simulink model "FaultCheck"  (R2022b)
settings: Solver=FixedStepAuto  StartTime=0.0  StopTime=10  FixedStep=1  RelTol=1e-3
undefined symbols (not defined in the file): C_Flt_IGBTULowerTempConfirmTh_u16, C_Flt_IGBTULowerTempDiagEn_b, C_Flt_IGBTULowerTempErrCode_u16, C_Flt_IGBTULowerTempPowerCoeff, C_Flt_IGBTULowerTempRecoveryTh_u16, C_Flt_IGBTULowerTempRecTh_s32, C_Flt_IGBTULowerTempTrigTh_s32, C_Flt_IGBTUOverTempConfirmTh_u16, C_Flt_IGBTUOverTempDiagEn_b, C_Flt_IGBTUOverTempErrCode_u16, C_Flt_IGBTUOverTempRecoveryTh_u16, C_Flt_IGBTUOverTempRecTh_s32, C_Flt_IGBTUOverTempTrigTh_s32, C_Flt_IGBTVLowerTempConfirmTh_u16, C_Flt_IGBTVLowerTempDiagEn_b, C_Flt_IGBTVLowerTempErrCode_u16, C_Flt_IGBTVLowerTempPowerCoeff, C_Flt_IGBTVLowerTempRecoveryTh_u16, C_Flt_IGBTVLowerTempRecTh_s32, C_Flt_IGBTVLowerTempTrigTh_s32, C_Flt_IGBTVOverTempConfirmTh_u16, C_Flt_IGBTVOverTempDiagEn_b, C_Flt_IGBTVOverTempErrCode_u16, C_Flt_IGBTVOverTempRecoveryTh_u16, C_Flt_IGBTVOverTempRecTh_s32, C_Flt_IGBTVOverTempTrigTh_s32, C_Flt_IGBTWLowerTempConfirmTh_u16, C_Flt_IGBTWLowerTempDiagEn_b, C_Flt_IGBTWLowerTempErrCode_u16, C_Flt_IGBTWLowerTempPowerCoeff, C_Flt_IGBTWLowerTempRecoveryTh_u16, C_Flt_IGBTWLowerTempRecTh_s32, C_Flt_IGBTWLowerTempTrigTh_s32, C_Flt_IGBTWOverTempConfirmTh_u16, C_Flt_IGBTWOverTempDiagEn_b, C_Flt_IGBTWOverTempErrCode_u16, C_Flt_IGBTWOverTempRecoveryTh_u16, C_Flt_IGBTWOverTempRecTh_s32, C_Flt_IGBTWOverTempTrigTh_s32, C_Flt_IuOCConfirmTh_u16, C_Flt_IuOCDiagEn_b, C_Flt_IuOCErrCode_u16, C_Flt_IuOCNegLimit_s32, C_Flt_IuOCPosLimit_s32, C_Flt_IuOCRecoveryTh_u16, C_Flt_IuZeroDriftDiagEn_b, C_Flt_IuZeroDriftErrCode_u16, C_Flt_IvOCConfirmTh_u16, C_Flt_IvOCDiagEn_b, C_Flt_IvOCErrCode_u16, C_Flt_IvOCNegLimit_s32, C_Flt_IvOCPosLimit_s32, C_Flt_IvOCRecoveryTh_u16, C_Flt_IvZeroDriftDiagEn_b, C_Flt_IvZeroDriftErrCode_u16, C_Flt_IwOCConfirmTh_u16, C_Flt_IwOCDiagEn_b, C_Flt_IwOCErrCode_u16, C_Flt_IwOCNegLimit_s32, C_Flt_IwOCPosLimit_s32 ... (+196)
libraries: YS_UserDefined_Library x21, simulink x5
(part 6 of 11)

== system FaultCheck/FaultDiagnose/UdcLowerTwoDiag/Diagnose/Disable ==
  Action Port : ActionPort  ActionPortLabel=if(u1 == 0)
  Constant : Constant  Value=C_Flt_NoErr_b
  UdcLowerTwoFltDeb : Outport
  wires:
  Constant/1 -> UdcLowerTwoFltDeb/1

== system FaultCheck/FaultDiagnose/UdcLowerTwoDiag/Diagnose/NormalDiag ==
  Udc : Inport
  Parameter : Inport  Port=2
  Action Port : ActionPort  ActionPortLabel=else
  Bus Selector : BusSelector  OutputSignals=UdcLowerTwoConfirmTh,UdcLowerTwoRecoveryTh,UdcLowerTwoTrigTh,UdcLowerTwoRecTh
  DebounceRecInTwo : YS_UserDefined_Library/Fault/DebounceRecInTwo  SystemSampleTime=-1  VariantActivationTime=update diagram  Latency=0  AutoFrameSizeCalculation=off
      settings: SourceProductName=YS
  Relational Operator : RelationalOperator  Operator=>  OutDataTypeStr=boolean  RndMeth=Simplest  InputSameDT=off
  Relational Operator1 : RelationalOperator  Operator=>  OutDataTypeStr=boolean  RndMeth=Simplest  InputSameDT=off
  Signal Copy : SignalConversion  OverrideOpt=off
  UdcLowerTwoFltDeb : Outport
  wires:
  Parameter/1 -> Bus Selector/1
  Bus Selector/1 -> DebounceRecInTwo/1  "<UdcLowerTwoConfirmTh>"
  Bus Selector/2 -> DebounceRecInTwo/2  "<UdcLowerTwoRecoveryTh>"
  DebounceRecInTwo/1 -> Signal Copy/1  "M_Flt_UdcLowerTwoFltFlgDeb_b"
  Relational Operator/1 -> DebounceRecInTwo/3  "M_Flt_UdcLowerTwoFltFlgUnDeb_b"
  Signal Copy/1 -> UdcLowerTwoFltDeb/1
  Bus Selector/3 -> Relational Operator/1  "<UdcLowerTwoTrigTh>"
  Udc/1 -> Relational Operator/2, Relational Operator1/1
  Bus Selector/4 -> Relational Operator1/2  "<UdcLowerTwoRecTh>"
  Relational Operator1/1 -> DebounceRecInTwo/4  "M_Flt_UdcLowerTwoRecFlgUnDeb_b"

== system FaultCheck/FaultDiagnose/UdcLowerTwoDiag/FaultLevelDeter/LowerTwo ==
  FaultLevel : Inport
  Action Port : ActionPort  ActionPortLabel=else
  UdcLowerTwoFltLevel : Outport
  wires:
  FaultLevel/1 -> UdcLowerTwoFltLevel/1

== system FaultCheck/FaultDiagnose/UdcLowerTwoDiag/FaultLevelDeter/Normal ==
  Action Port : ActionPort  ActionPortLabel=if(u1 == 0)
  Constant : Constant  Value=C_Flt_LevelZero_u8
  UdcLowerTwoFltLevel : Outport
  wires:
  Constant/1 -> UdcLowerTwoFltLevel/1

== system FaultCheck/FaultDiagnose/UdcLowerTwoDiag/PowerReductionCoeffDeter/If Action Subsystem ==
  Action Port : ActionPort  ActionPortLabel=if(u1 < 2)
  Constant : Constant  Value=C_Flt_PowerCoeffOne_s32
  Coeff : Outport
  wires:
  Constant/1 -> Coeff/1

== system FaultCheck/FaultDiagnose/UdcLowerTwoDiag/PowerReductionCoeffDeter/If Action Subsystem1 ==
  PowerCoeff : Inport
  Action Port : ActionPort  ActionPortLabel=elseif(u1 == 2)
  Coeff : Outport
  wires:
  PowerCoeff/1 -> Coeff/1

== system FaultCheck/FaultDiagnose/UdcLowerTwoDiag/PowerReductionCoeffDeter/If Action Subsystem2 ==
  Action Port : ActionPort  ActionPortLabel=else
  Constant : Constant  Value=C_Flt_PowerCoeffZero_s32
  Coeff : Outport
  wires:
  Constant/1 -> Coeff/1

== system FaultCheck/FaultDiagnose/UdcOverOneDiag/Diagnose/Disable ==
  Action Port : ActionPort  ActionPortLabel=if(u1 == 0)
  Constant : Constant  Value=C_Flt_NoErr_b
  UdcOverOneFltDeb : Outport
  wires:
  Constant/1 -> UdcOverOneFltDeb/1

== system FaultCheck/FaultDiagnose/UdcOverOneDiag/Diagnose/NormalDiag ==
  Udc : Inport
  Parameter : Inport  Port=2
  Action Port : ActionPort  ActionPortLabel=else
  Bus Selector : BusSelector  OutputSignals=UdcOverOneConfirmTh,UdcOverOneRecoveryTh,UdcOverOneTrigTh,UdcOverOneRecTh
  DebounceRecInTwo : YS_UserDefined_Library/Fault/DebounceRecInTwo  SystemSampleTime=-1  VariantActivationTime=update diagram  Latency=0  AutoFrameSizeCalculation=off
      settings: SourceProductName=YS
  Relational Operator : RelationalOperator  Operator=<  OutDataTypeStr=boolean  RndMeth=Simplest  InputSameDT=off
  Relational Operator1 : RelationalOperator  Operator=<  OutDataTypeStr=boolean  RndMeth=Simplest  InputSameDT=off
  Signal Copy : SignalConversion  OverrideOpt=off
  UdcOverOneFltDeb : Outport
  wires:
  Parameter/1 -> Bus Selector/1
  Bus Selector/1 -> DebounceRecInTwo/1  "<UdcOverOneConfirmTh>"
  Bus Selector/2 -> DebounceRecInTwo/2  "<UdcOverOneRecoveryTh>"
  DebounceRecInTwo/1 -> Signal Copy/1  "M_Flt_UdcOverOneFltFlgDeb_b"
  Relational Operator/1 -> DebounceRecInTwo/3  "M_Flt_UdcOverOneFltFlgUnDeb_b"
  Signal Copy/1 -> UdcOverOneFltDeb/1
  Bus Selector/3 -> Relational Operator/1  "<UdcOverOneTrigTh>"
  Udc/1 -> Relational Operator1/1, Relational Operator/2
  Bus Selector/4 -> Relational Operator1/2  "<UdcOverOneRecTh>"
  Relational Operator1/1 -> DebounceRecInTwo/4  "M_Flt_UdcOverOneRecFlgUnDeb_b"

== system FaultCheck/FaultDiagnose/UdcOverOneDiag/FaultLevelDeter/Normal ==
  Action Port : ActionPort  ActionPortLabel=if(u1 == 0)
  Constant : Constant  Value=C_Flt_LevelZero_u8
  UdcOverOneFltLevel : Outport
  wires:
  Constant/1 -> UdcOverOneFltLevel/1

== system FaultCheck/FaultDiagnose/UdcOverOneDiag/FaultLevelDeter/OverOne ==
  FaultLevel : Inport
  Action Port : ActionPort  ActionPortLabel=else
  UdcOverOneFltLevel : Outport
  wires:
  FaultLevel/1 -> UdcOverOneFltLevel/1

== system FaultCheck/FaultDiagnose/UdcOverOneDiag/PowerReductionCoeffDeter/If Action Subsystem ==
  Action Port : ActionPort  ActionPortLabel=if(u1 < 2)
  Constant : Constant  Value=C_Flt_PowerCoeffOne_s32
  Coeff : Outport
  wires:
  Constant/1 -> Coeff/1

== system FaultCheck/FaultDiagnose/UdcOverOneDiag/PowerReductionCoeffDeter/If Action Subsystem1 ==
  PowerCoeff : Inport
  Action Port : ActionPort  ActionPortLabel=elseif(u1 == 2)
  Coeff : Outport
  wires:
  PowerCoeff/1 -> Coeff/1

== system FaultCheck/FaultDiagnose/UdcOverOneDiag/PowerReductionCoeffDeter/If Action Subsystem2 ==
  Action Port : ActionPort  ActionPortLabel=else
  Constant : Constant  Value=C_Flt_PowerCoeffZero_s32
  Coeff : Outport
  wires:
  Constant/1 -> Coeff/1

== system FaultCheck/FaultDiagnose/UdcOverTwoDiag/Diagnose/Disable ==
  Action Port : ActionPort  ActionPortLabel=if(u1 == 0)
  Constant : Constant  Value=C_Flt_NoErr_b
  UdcOverTwoFltDeb : Outport
  wires:
  Constant/1 -> UdcOverTwoFltDeb/1

== system FaultCheck/FaultDiagnose/UdcOverTwoDiag/Diagnose/NormalDiag ==
  Udc : Inport
  Parameter : Inport  Port=2
  Action Port : ActionPort  ActionPortLabel=else
  Bus Selector : BusSelector  OutputSignals=UdcOverTwoConfirmTh,UdcOverTwoRecoveryTh,UdcOverTwoTrigTh
  DebounceUnRec1 : YS_UserDefined_Library/Fault/DebounceUnRec  SystemSampleTime=-1  VariantActivationTime=update diagram  Latency=0  AutoFrameSizeCalculation=off
      settings: SourceProductName=YS
  Relational Operator : RelationalOperator  Operator=<  OutDataTypeStr=boolean  RndMeth=Simplest  InputSameDT=off
  Signal Copy : SignalConversion  OverrideOpt=off
  UdcOverTwoFltDeb : Outport
  wires:
  Parameter/1 -> Bus Selector/1
  Bus Selector/1 -> DebounceUnRec1/1  "<UdcOverTwoConfirmTh>"
  Bus Selector/2 -> DebounceUnRec1/2  "<UdcOverTwoRecoveryTh>"
  DebounceUnRec1/1 -> Signal Copy/1  "M_Flt_UdcOverTwoFltFlgDeb_b"
  Relational Operator/1 -> DebounceUnRec1/3  "M_Flt_UdcOverTwoFltFlgUnDeb_b"
  Signal Copy/1 -> UdcOverTwoFltDeb/1
  Bus Selector/3 -> Relational Operator/1  "<UdcOverTwoTrigTh>"
  Udc/1 -> Relational Operator/2

== system FaultCheck/FaultDiagnose/UdcOverTwoDiag/FaultLevelDeter/Normal ==
  Action Port : ActionPort  ActionPortLabel=if(u1 == 0)
  Constant : Constant  Value=C_Flt_LevelZero_u8
  UdcOverTwoFltLevel : Outport
  wires:
  Constant/1 -> UdcOverTwoFltLevel/1

== system FaultCheck/FaultDiagnose/UdcOverTwoDiag/FaultLevelDeter/OverTwo ==
  FaultLevel : Inport
  Action Port : ActionPort  ActionPortLabel=else
  UdcOverTwoFltLevel : Outport
  wires:
  FaultLevel/1 -> UdcOverTwoFltLevel/1

== system FaultCheck/FaultDiagnose/UdcOverTwoDiag/PowerReductionCoeffDeter/If Action Subsystem ==
  Action Port : ActionPort  ActionPortLabel=if(u1 < 2)
  Constant : Constant  Value=C_Flt_PowerCoeffOne_s32
  Coeff : Outport
  wires:
  Constant/1 -> Coeff/1

== system FaultCheck/FaultDiagnose/UdcOverTwoDiag/PowerReductionCoeffDeter/If Action Subsystem1 ==
  PowerCoeff : Inport
  Action Port : ActionPort  ActionPortLabel=elseif(u1 == 2)
  Coeff : Outport
  wires:
  PowerCoeff/1 -> Coeff/1

== system FaultCheck/FaultDiagnose/UdcOverTwoDiag/PowerReductionCoeffDeter/If Action Subsystem2 ==
  Action Port : ActionPort  ActionPortLabel=else
  Constant : Constant  Value=C_Flt_PowerCoeffZero_s32
  Coeff : Outport
  wires:
  Constant/1 -> Coeff/1

== system FaultCheck/FltCheck/Determination/Detection Criteria/Determination ==
  Condition : Inport
  EQ : Inport  Port=2
  GT : Inport  Port=3
  LT : Inport  Port=4
  NEQ : Inport  Port=5
  Multiport Switch : MultiPortSwitch  Inputs=4  SaturateOnIntegerOverflow=off  InputSameDT=off
  Fail : Outport
  wires:
  EQ/1 -> Multiport Switch/2
  GT/1 -> Multiport Switch/3
  LT/1 -> Multiport Switch/4
  NEQ/1 -> Multiport Switch/5
  Condition/1 -> Multiport Switch/1
  Multiport Switch/1 -> Fail/1

== system FaultCheck/FltCheck/Determination/Detection Criteria/Equal ==
  FltSrc : Inport
  FltTh : Inport  Port=2
  Constant : Constant  OutDataTypeStr=boolean
  Constant1 : Constant  Value=0  OutDataTypeStr=boolean
  Relational Operator : RelationalOperator  Operator===  OutDataTypeStr=boolean  RndMeth=Simplest  InputSameDT=off
  Switch : Switch  Criteria=u2 ~= 0  SaturateOnIntegerOverflow=off  InputSameDT=off
  EQ : Outport
  wires:
  FltSrc/1 -> Relational Operator/1
  FltTh/1 -> Relational Operator/2
  Relational Operator/1 -> Switch/2
  Constant/1 -> Switch/1
  Constant1/1 -> Switch/3
  Switch/1 -> EQ/1

== system FaultCheck/FltCheck/Determination/Detection Criteria/Lower ==
  FltSrc : Inport
  FltTh : Inport  Port=2
  Constant : Constant  OutDataTypeStr=boolean
  Constant1 : Constant  Value=0  OutDataTypeStr=boolean
  Relational Operator : RelationalOperator  Operator=<  OutDataTypeStr=boolean  RndMeth=Simplest  InputSameDT=off
  Switch : Switch  Criteria=u2 ~= 0  SaturateOnIntegerOverflow=off  InputSameDT=off
  LT : Outport
  wires:
  FltSrc/1 -> Relational Operator/1
  FltTh/1 -> Relational Operator/2
  Relational Operator/1 -> Switch/2
  Constant/1 -> Switch/1
  Constant1/1 -> Switch/3
  Switch/1 -> LT/1

== system FaultCheck/FltCheck/Determination/Detection Criteria/NotEqual ==
  FltSrc : Inport
  FltTh : Inport  Port=2
  Constant : Constant  OutDataTypeStr=boolean
  Constant1 : Constant  Value=0  OutDataTypeStr=boolean
  Relational Operator : RelationalOperator  Operator=~=  OutDataTypeStr=boolean  RndMeth=Simplest  InputSameDT=off
  Switch : Switch  Criteria=u2 ~= 0  SaturateOnIntegerOverflow=off  InputSameDT=off
  NEQ : Outport
  wires:
  Switch/1 -> NEQ/1
  Constant1/1 -> Switch/3
  Constant/1 -> Switch/1
  Relational Operator/1 -> Switch/2
  FltTh/1 -> Relational Operator/2
  FltSrc/1 -> Relational Operator/1

== system FaultCheck/FltCheck/Determination/Detection Criteria/Overflow ==
  FltSrc : Inport
  FltTh : Inport  Port=2
  Constant : Constant  OutDataTypeStr=boolean
  Constant1 : Constant  Value=0  OutDataTypeStr=boolean
  Relational Operator : RelationalOperator  Operator=>  OutDataTypeStr=boolean  RndMeth=Simplest  InputSameDT=off
  Switch : Switch  Criteria=u2 ~= 0  SaturateOnIntegerOverflow=off  InputSameDT=off
  GT : Outport
  wires:
  Switch/1 -> GT/1
  Constant1/1 -> Switch/3
  Constant/1 -> Switch/1
  Relational Operator/1 -> Switch/2
  FltTh/1 -> Relational Operator/2
  FltSrc/1 -> Relational Operator/1

== system FaultCheck/FaultDiag_HighTask_100us/FltDetn/CurrentSensorDetn/Flt_CurrentSensorDetn/ErrCode ==
  note: SWFD--ComReq-01-13
  ErrDetnFlgOut : Inport
  ErrCode : Inport  Port=2
  If : If  IfExpression=u1==0
  If Action Subsystem : Subsystem  TreatAsAtomicUnit=on
  If Action Subsystem1 : Subsystem  TreatAsAtomicUnit=on
  wires:
  ErrCode/1 -> If Action Subsystem1/1(ErrCod)
  If/1 -> If Action Subsystem/Action
  If/2 -> If Action Subsystem1/Action
  ErrDetnFlgOut/1 -> If/1

== system FaultCheck/FaultDiag_HighTask_100us/FltDetn/CurrentSensorDetn/Flt_CurrentSensorDetn/ErrDetn ==
  InputVal : Inport
  EnabDetn : Inport  Port=2
  ActvnDetn : Inport  Port=3
  ErrDeb : Inport  Port=4
  AND1 : Logic  AllPortsSameDT=off  OutDataTypeStr=boolean
  Constant10 : Constant  Value=FLT_ON
  Constant9 : Constant  Value=FLT_ON
  If : If  IfExpression=u1 == 0
  If Action Subsystem : Subsystem  TreatAsAtomicUnit=on
  If Action Subsystem1 : Subsystem  TreatAsAtomicUnit=on
  Merge : Merge
  Relational Operator3 : RelationalOperator  Operator===  OutDataTypeStr=boolean  RndMeth=Simplest  InputSameDT=off
  Relational Operator4 : RelationalOperator  Operator===  OutDataTypeStr=boolean  RndMeth=Simplest  InputSameDT=off
  Flt_CurrentSensorErrFlg : Outport
  wires:
  InputVal/1 -> If Action Subsystem1/1(InputVal)
  ActvnDetn/1 -> Relational Operator3/1
  Constant10/1 -> Relational Operator4/1
  EnabDetn/1 -> Relational Operator4/2
  Relational Operator3/1 -> AND1/1
  Constant9/1 -> Relational Operator3/2
  Relational Operator4/1 -> AND1/2
  AND1/1 -> If/1
  If/1 -> If Action Subsystem/Action
  If/2 -> If Action Subsystem1/Action
  If Action Subsystem1/1(Out1) -> Merge/2
  If Action Subsystem/1(Out1) -> Merge/1
  Merge/1 -> Flt_CurrentSensorErrFlg/1
  ErrDeb/1 -> If Action Subsystem1/2(ErrDeb)

== system FaultCheck/FaultDiag_HighTask_100us/FltDetn/CurrentSensorDetn/Flt_CurrentSensorDetn/FltLvl ==
  note: SWFD--ComReq-01-09
      | SWFD--ComReq-01-10
      | SWFD--ComReq-01-11
      | SWFD--ComReq-01-12
  ErrDetnFlgOut : Inport
  FltLvl : Inport  Port=2
  If : If  IfExpression=u1==0
  If Action Subsystem : Subsystem  TreatAsAtomicUnit=on
  If Action Subsystem1 : Subsystem  TreatAsAtomicUnit=on
  Merge : Merge
  Flt_CurrentSensorFltLvl : Outport
  wires:
  If Action Subsystem/1(ValOut) -> Merge/1
  Merge/1 -> Flt_CurrentSensorFltLvl/1  "Flt_CurrentSensorFltLvl"
  If/1 -> If Action Subsystem/Action
  If/2 -> If Action Subsystem1/Action
  ErrDetnFlgOut/1 -> If/1
  FltLvl/1 -> If Action Subsystem1/1(In)
  If Action Subsystem1/1(ValOut) -> Merge/2

== system FaultCheck/FaultDiag_HighTask_100us/FltDetn/CurrentSensorDetn/Flt_CurrentSensorDetn/Power Reduction Coefficient ==
  note: SWFD--ComReq-01-06
      | SWFD--ComReq-01-07
      | SWFD--ComReq-01-08
      | SWFD--ComReq-01-09
  FltLvlOut : Inport
  PowRecCoef : Inport  Port=2
  If : If  IfExpression=u1<2  ElseIfExpressions=u1==2
  If Action Subsystem : Subsystem  TreatAsAtomicUnit=on
  If Action Subsystem1 : Subsystem  TreatAsAtomicUnit=on
  If Action Subsystem2 : Subsystem  TreatAsAtomicUnit=on
  Merge : Merge  Inputs=3
  Flt_CurrentSensorPowRecCoefOut : Outport
  wires:
  If/1 -> If Action Subsystem/Action
  If Action Subsystem2/1(PowRecCoefOut) -> Merge/3
  If/3 -> If Action Subsystem2/Action
  FltLvlOut/1 -> If/1
  PowRecCoef/1 -> If Action Subsystem1/1(PowRecCoef)
  If Action Subsystem1/1(PowRecCoefOut) -> Merge/2
  If Action Subsystem/1(PowRecCoefOut) -> Merge/1
  Merge/1 -> Flt_CurrentSensorPowRecCoefOut/1  "Flt_CurrentSensorPowRecCoefOut"
  If/2 -> If Action Subsystem1/Action

== system FaultCheck/FaultDiag_HighTask_100us/FltDetn/CurrentSensorDetn/Flt_CurrentSensorDetn/Subsystem ==
  note: SWFD--ComReq-01-14
  Flt_CurrentSensorErrDetnFlg : Inport
  IPC_IuRaw_A : Inport  Port=2
  IPC_IvRaw_A : Inport  Port=3
  Constant : Constant  Value=Flt_IuCurrentSensorSubValue
  Constant1 : Constant  Value=Flt_IvCurrentSensorSubValue
  Switch : Switch  Criteria=u2 > Threshold  SaturateOnIntegerOverflow=off  InputSameDT=off
  Switch1 : Switch  Criteria=u2 > Threshold  SaturateOnIntegerOverflow=off  InputSameDT=off
  Flt_IuCurrentSensorFin : Outport
  Flt_IvCurrentSensorFin : Outport  Port=2
  wires:
  Switch1/1 -> Flt_IvCurrentSensorFin/1
  Flt_CurrentSensorErrDetnFlg/1 -> Switch/2, Switch1/2
  Constant1/1 -> Switch1/1
  IPC_IvRaw_A/1 -> Switch1/3
  Constant/1 -> Switch/1
  Switch/1 -> Flt_IuCurrentSensorFin/1
  IPC_IuRaw_A/1 -> Switch/3

== system FaultCheck/FaultDiag_HighTask_100us/FltDetn/CurrentZeroDrfDetn/CurrZeroDrfDetn/ErrCode1 ==
  ErrDetnFlgOut : Inport
  ErrCode : Inport  Port=2
  If : If  IfExpression=u1==0
  If Action Subsystem : Subsystem  TreatAsAtomicUnit=on
  If Action Subsystem1 : Subsystem  TreatAsAtomicUnit=on
  wires:
  ErrDetnFlgOut/1 -> If/1
  If/2 -> If Action Subsystem1/Action
  If/1 -> If Action Subsystem/Action
  ErrCode/1 -> If Action Subsystem1/1(ErrCod)

== system FaultCheck/FaultDiag_HighTask_100us/FltDetn/CurrentZeroDrfDetn/CurrZeroDrfDetn/ErrDetn ==
  InputVal : Inport
  EnabDetn : Inport  Port=2
  ActvnDetn : Inport  Port=3
  AND1 : Logic  AllPortsSameDT=off  OutDataTypeStr=boolean
  Constant10 : Constant  Value=FLT_ON
  Constant9 : Constant  Value=FLT_ON
  If : If  IfExpression=u1 == 0
  If Action Subsystem : Subsystem  TreatAsAtomicUnit=on
  If Action Subsystem1 : Subsystem  TreatAsAtomicUnit=on
  Merge : Merge
  Relational Operator3 : RelationalOperator  Operator===  OutDataTypeStr=boolean  RndMeth=Simplest  InputSameDT=off
  Relational Operator4 : RelationalOperator  Operator===  OutDataTypeStr=boolean  RndMeth=Simplest  InputSameDT=off
  Flt_CurrZeroDrfErrFlg : Outport
  wires:
  ActvnDetn/1 -> Relational Operator3/1
  Constant10/1 -> Relational Operator4/1
  EnabDetn/1 -> Relational Operator4/2
  Relational Operator3/1 -> AND1/1
  Constant9/1 -> Relational Operator3/2
  Relational Operator4/1 -> AND1/2
  AND1/1 -> If/1
  If/1 -> If Action Subsystem/Action
  If/2 -> If Action Subsystem1/Action
  If Action Subsystem1/1(Out1) -> Merge/2
  If Action Subsystem/1(Out1) -> Merge/1
  Merge/1 -> Flt_CurrZeroDrfErrFlg/1  "Flt_CurrZeroDrfErrFlg"
  InputVal/1 -> If Action Subsystem1/1(InputVal)

== system FaultCheck/FaultDiag_HighTask_100us/FltDetn/CurrentZeroDrfDetn/CurrZeroDrfDetn/FltLvl ==
  ErrDetnFlgOut : Inport
  FltLvl : Inport  Port=2
  If : If  IfExpression=u1==0
  If Action Subsystem : Subsystem  TreatAsAtomicUnit=on
  If Action Subsystem1 : Subsystem  TreatAsAtomicUnit=on
  Merge : Merge
  Flt_CurrZeroDrfFltLvl : Outport
  wires:
  If Action Subsystem/1(ValOut) -> Merge/1
  Merge/1 -> Flt_CurrZeroDrfFltLvl/1  "Flt_CurrZeroDrfFltLv"
  If/1 -> If Action Subsystem/Action
  If/2 -> If Action Subsystem1/Action
  ErrDetnFlgOut/1 -> If/1
  FltLvl/1 -> If Action Subsystem1/1(In)
  If Action Subsystem1/1(ValOut) -> Merge/2

== system FaultCheck/FaultDiag_HighTask_100us/FltDetn/CurrentZeroDrfDetn/CurrZeroDrfDetn/Power Reduction Coefficient ==
  FltLvlOut : Inport
  PowRecCoef : Inport  Port=2
  If : If  IfExpression=u1<2  ElseIfExpressions=u1==2
  If Action Subsystem : Subsystem  TreatAsAtomicUnit=on
  If Action Subsystem1 : Subsystem  TreatAsAtomicUnit=on
  If Action Subsystem2 : Subsystem  TreatAsAtomicUnit=on
  Merge : Merge  Inputs=3
  Flt_CurrZeroDrfPowRecCoefOut : Outport
  wires:
  If/2 -> If Action Subsystem1/Action
  Merge/1 -> Flt_CurrZeroDrfPowRecCoefOut/1  "Flt_CurrZeroDrfPowRecCoefOut"
  If Action Subsystem/1(PowRecCoefOut) -> Merge/1
  If Action Subsystem1/1(PowRecCoefOut) -> Merge/2
  PowRecCoef/1 -> If Action Subsystem1/1(PowRecCoef)
  FltLvlOut/1 -> If/1
  If/3 -> If Action Subsystem2/Action
  If Action Subsystem2/1(PowRecCoefOut) -> Merge/3
  If/1 -> If Action Subsystem/Action

== system FaultCheck/FaultDiag_HighTask_100us/FltDetn/DriveUdcDetn/DriveUdcDetn/ErrCode ==
  ErrDetnFlgOut : Inport
  ErrCode : Inport  Port=2
  If : If  IfExpression=u1==0
  If Action Subsystem : Subsystem  TreatAsAtomicUnit=on
  If Action Subsystem1 : Subsystem  TreatAsAtomicUnit=on
  wires:
  ErrDetnFlgOut/1 -> If/1
  If/2 -> If Action Subsystem1/Action
  If/1 -> If Action Subsystem/Action
  ErrCode/1 -> If Action Subsystem1/1(ErrCod)

== system FaultCheck/FaultDiag_HighTask_100us/FltDetn/DriveUdcDetn/DriveUdcDetn/ErrDetn ==
  InputVal : Inport
  EnabDetn : Inport  Port=2
  ActvnDetn : Inport  Port=3
  ErrDeb : Inport  Port=4
  AND1 : Logic  AllPortsSameDT=off  OutDataTypeStr=boolean
  Constant10 : Constant  Value=FLT_ON
  Constant9 : Constant  Value=FLT_ON
  If : If  IfExpression=u1 == 0
  If Action Subsystem : Subsystem  TreatAsAtomicUnit=on
  If Action Subsystem1 : Subsystem  TreatAsAtomicUnit=on
  Merge : Merge
  Relational Operator3 : RelationalOperator  Operator===  OutDataTypeStr=boolean  RndMeth=Simplest  InputSameDT=off
  Relational Operator4 : RelationalOperator  Operator===  OutDataTypeStr=boolean  RndMeth=Simplest  InputSameDT=off
  Flt_DriveUdcErrFlg : Outport
  wires:
  ErrDeb/1 -> If Action Subsystem1/2(ErrDeb)
  Merge/1 -> Flt_DriveUdcErrFlg/1  "Flt_DriveUdcErrFlg"
  If Action Subsystem/1(Out1) -> Merge/1
  If Action Subsystem1/1(Out1) -> Merge/2
  If/2 -> If Action Subsystem1/Action
  If/1 -> If Action Subsystem/Action
  AND1/1 -> If/1
  Relational Operator4/1 -> AND1/2
  Constant9/1 -> Relational Operator3/2
  Relational Operator3/1 -> AND1/1
  EnabDetn/1 -> Relational Operator4/2
  Constant10/1 -> Relational Operator4/1
  ActvnDetn/1 -> Relational Operator3/1
  InputVal/1 -> If Action Subsystem1/1(InputVal)

== system FaultCheck/FaultDiag_HighTask_100us/FltDetn/DriveUdcDetn/DriveUdcDetn/FltLvl ==
  ErrDetnFlgOut : Inport
  FltLvl : Inport  Port=2
  If : If  IfExpression=u1==0
  If Action Subsystem : Subsystem  TreatAsAtomicUnit=on
  If Action Subsystem1 : Subsystem  TreatAsAtomicUnit=on
  Merge : Merge
  Flt_DriveUdcFltLvl : Outport
  wires:
  If Action Subsystem1/1(ValOut) -> Merge/2
  FltLvl/1 -> If Action Subsystem1/1(In)
  ErrDetnFlgOut/1 -> If/1
  If/2 -> If Action Subsystem1/Action
  If/1 -> If Action Subsystem/Action
  Merge/1 -> Flt_DriveUdcFltLvl/1  "Flt_DriveUdcFltLvl"
  If Action Subsystem/1(ValOut) -> Merge/1

== system FaultCheck/FaultDiag_HighTask_100us/FltDetn/DriveUdcDetn/DriveUdcDetn/Power Reduction Coefficient ==
  FltLvlOut : Inport
  PowRecCoef : Inport  Port=2
  If : If  IfExpression=u1<2  ElseIfExpressions=u1==2
  If Action Subsystem : Subsystem  TreatAsAtomicUnit=on
  If Action Subsystem1 : Subsystem  TreatAsAtomicUnit=on
  If Action Subsystem2 : Subsystem  TreatAsAtomicUnit=on
  Merge : Merge  Inputs=3
  Flt_DriveUdcPowRecCoefOut : Outport
  wires:
  If/2 -> If Action Subsystem1/Action
  Merge/1 -> Flt_DriveUdcPowRecCoefOut/1  "Flt_DriveUdcPowRecCoefOut"
  If Action Subsystem/1(PowRecCoefOut) -> Merge/1
  If Action Subsystem1/1(PowRecCoefOut) -> Merge/2
  PowRecCoef/1 -> If Action Subsystem1/1(PowRecCoef)
  FltLvlOut/1 -> If/1
  If/3 -> If Action Subsystem2/Action
  If Action Subsystem2/1(PowRecCoefOut) -> Merge/3
  If/1 -> If Action Subsystem/Action

== system FaultCheck/FaultDiag_HighTask_100us/FltDetn/Drive_H_Detn/Drive_H_Detn/ErrCode ==
  ErrDetnFlgOut : Inport
  ErrCode : Inport  Port=2
  If : If  IfExpression=u1==0
  If Action Subsystem : Subsystem  TreatAsAtomicUnit=on
  If Action Subsystem1 : Subsystem  TreatAsAtomicUnit=on
  wires:
  ErrDetnFlgOut/1 -> If/1
  If/2 -> If Action Subsystem1/Action
  If/1 -> If Action Subsystem/Action
  ErrCode/1 -> If Action Subsystem1/1(ErrCod)

== system FaultCheck/FaultDiag_HighTask_100us/FltDetn/Drive_H_Detn/Drive_H_Detn/ErrDetn ==
  InputVal : Inport
  EnabDetn : Inport  Port=2
  ActvnDetn : Inport  Port=3
  ErrDeb : Inport  Port=4
  AND1 : Logic  AllPortsSameDT=off  OutDataTypeStr=boolean
  Constant10 : Constant  Value=FLT_ON
  Constant9 : Constant  Value=FLT_ON
  If : If  IfExpression=u1 == 0
  If Action Subsystem : Subsystem  TreatAsAtomicUnit=on
  If Action Subsystem1 : Subsystem  TreatAsAtomicUnit=on
  Merge : Merge
  Relational Operator3 : RelationalOperator  Operator===  OutDataTypeStr=boolean  RndMeth=Simplest  InputSameDT=off
  Relational Operator4 : RelationalOperator  Operator===  OutDataTypeStr=boolean  RndMeth=Simplest  InputSameDT=off
  Flt_Drive_H_ErrFlg : Outport
  wires:
  ErrDeb/1 -> If Action Subsystem1/2(ErrDeb)
  Merge/1 -> Flt_Drive_H_ErrFlg/1  "Flt_Drive_H_ErrFlg"
  If Action Subsystem/1(Out1) -> Merge/1
  If Action Subsystem1/1(Out1) -> Merge/2
  If/2 -> If Action Subsystem1/Action
  If/1 -> If Action Subsystem/Action
  AND1/1 -> If/1
  Relational Operator4/1 -> AND1/2
  Constant9/1 -> Relational Operator3/2
  Relational Operator3/1 -> AND1/1
  EnabDetn/1 -> Relational Operator4/2
  Constant10/1 -> Relational Operator4/1
  ActvnDetn/1 -> Relational Operator3/1
  InputVal/1 -> If Action Subsystem1/1(InputVal)

== system FaultCheck/FaultDiag_HighTask_100us/FltDetn/Drive_H_Detn/Drive_H_Detn/FltLvl ==
  ErrDetnFlgOut : Inport
  FltLvl : Inport  Port=2
  If : If  IfExpression=u1==0
  If Action Subsystem : Subsystem  TreatAsAtomicUnit=on
  If Action Subsystem1 : Subsystem  TreatAsAtomicUnit=on
  Merge : Merge
  Flt_Drive_H_FltLvl : Outport
  wires:
  If Action Subsystem1/1(ValOut) -> Merge/2
  FltLvl/1 -> If Action Subsystem1/1(In)
  ErrDetnFlgOut/1 -> If/1
  If/2 -> If Action Subsystem1/Action
  If/1 -> If Action Subsystem/Action
  Merge/1 -> Flt_Drive_H_FltLvl/1  "Flt_Drive_H_FltLvl"
  If Action Subsystem/1(ValOut) -> Merge/1

== system FaultCheck/FaultDiag_HighTask_100us/FltDetn/Drive_H_Detn/Drive_H_Detn/Power Reduction Coefficient ==
  FltLvlOut : Inport
  PowRecCoef : Inport  Port=2
  If : If  IfExpression=u1<2  ElseIfExpressions=u1==2
  If Action Subsystem : Subsystem  TreatAsAtomicUnit=on
  If Action Subsystem1 : Subsystem  TreatAsAtomicUnit=on
  If Action Subsystem2 : Subsystem  TreatAsAtomicUnit=on
  Merge : Merge  Inputs=3
  Flt_Drive_H_PowRecCoefOut : Outport
  wires:
  If/2 -> If Action Subsystem1/Action
  Merge/1 -> Flt_Drive_H_PowRecCoefOut/1  "Flt_Drive_H_PowRecCoefOut"
  If Action Subsystem/1(PowRecCoefOut) -> Merge/1
  If Action Subsystem1/1(PowRecCoefOut) -> Merge/2
  PowRecCoef/1 -> If Action Subsystem1/1(PowRecCoef)
  FltLvlOut/1 -> If/1
  If/3 -> If Action Subsystem2/Action
  If Action Subsystem2/1(PowRecCoefOut) -> Merge/3
  If/1 -> If Action Subsystem/Action

== system FaultCheck/FaultDiag_HighTask_100us/FltDetn/Drive_L_Detn/Drive_L_Detn/ErrCode ==
  ErrDetnFlgOut : Inport
  ErrCode : Inport  Port=2
  If : If  IfExpression=u1==0
  If Action Subsystem : Subsystem  TreatAsAtomicUnit=on
  If Action Subsystem1 : Subsystem  TreatAsAtomicUnit=on
  wires:
  ErrDetnFlgOut/1 -> If/1
  If/2 -> If Action Subsystem1/Action
  If/1 -> If Action Subsystem/Action
  ErrCode/1 -> If Action Subsystem1/1(ErrCod)

== system FaultCheck/FaultDiag_HighTask_100us/FltDetn/Drive_L_Detn/Drive_L_Detn/ErrDetn ==
  InputVal : Inport
  EnabDetn : Inport  Port=2
  ActvnDetn : Inport  Port=3
  ErrDeb : Inport  Port=4
  AND1 : Logic  AllPortsSameDT=off  OutDataTypeStr=boolean
  Constant10 : Constant  Value=FLT_ON
  Constant9 : Constant  Value=FLT_ON
  If : If  IfExpression=u1 == 0
  If Action Subsystem : Subsystem  TreatAsAtomicUnit=on
  If Action Subsystem1 : Subsystem  TreatAsAtomicUnit=on
  Merge : Merge
  Relational Operator3 : RelationalOperator  Operator===  OutDataTypeStr=boolean  RndMeth=Simplest  InputSameDT=off
  Relational Operator4 : RelationalOperator  Operator===  OutDataTypeStr=boolean  RndMeth=Simplest  InputSameDT=off
  Flt_Drive_L_ErrFlg : Outport
  wires:
  ErrDeb/1 -> If Action Subsystem1/2(ErrDeb)
  Merge/1 -> Flt_Drive_L_ErrFlg/1  "Flt_Drive_L_ErrFlg"
  If Action Subsystem/1(Out1) -> Merge/1
  If Action Subsystem1/1(Out1) -> Merge/2
  If/2 -> If Action Subsystem1/Action
  If/1 -> If Action Subsystem/Action
  AND1/1 -> If/1
  Relational Operator4/1 -> AND1/2
  Constant9/1 -> Relational Operator3/2
  Relational Operator3/1 -> AND1/1
  EnabDetn/1 -> Relational Operator4/2
  Constant10/1 -> Relational Operator4/1
  ActvnDetn/1 -> Relational Operator3/1
  InputVal/1 -> If Action Subsystem1/1(InputVal)

== system FaultCheck/FaultDiag_HighTask_100us/FltDetn/Drive_L_Detn/Drive_L_Detn/FltLvl ==
  ErrDetnFlgOut : Inport
  FltLvl : Inport  Port=2
  If : If  IfExpression=u1==0
  If Action Subsystem : Subsystem  TreatAsAtomicUnit=on
  If Action Subsystem1 : Subsystem  TreatAsAtomicUnit=on
  Merge : Merge
  Flt_Drive_L_FltLvl : Outport
  wires:
  If Action Subsystem1/1(ValOut) -> Merge/2
  FltLvl/1 -> If Action Subsystem1/1(In)
  ErrDetnFlgOut/1 -> If/1
  If/2 -> If Action Subsystem1/Action
  If/1 -> If Action Subsystem/Action
  Merge/1 -> Flt_Drive_L_FltLvl/1  "Flt_Drive_L_FltLvl"
  If Action Subsystem/1(ValOut) -> Merge/1

== system FaultCheck/FaultDiag_HighTask_100us/FltDetn/Drive_L_Detn/Drive_L_Detn/Power Reduction Coefficient ==
  FltLvlOut : Inport
  PowRecCoef : Inport  Port=2
  If : If  IfExpression=u1<2  ElseIfExpressions=u1==2
  If Action Subsystem : Subsystem  TreatAsAtomicUnit=on
  If Action Subsystem1 : Subsystem  TreatAsAtomicUnit=on
  If Action Subsystem2 : Subsystem  TreatAsAtomicUnit=on
  Merge : Merge  Inputs=3
  Flt_Drive_L_PowRecCoefOut : Outport
  wires:
  If/2 -> If Action Subsystem1/Action
  Merge/1 -> Flt_Drive_L_PowRecCoefOut/1  "Flt_Drive_L_PowRecCoefOut"
  If Action Subsystem/1(PowRecCoefOut) -> Merge/1
  If Action Subsystem1/1(PowRecCoefOut) -> Merge/2
  PowRecCoef/1 -> If Action Subsystem1/1(PowRecCoef)
  FltLvlOut/1 -> If/1
  If/3 -> If Action Subsystem2/Action
  If Action Subsystem2/1(PowRecCoefOut) -> Merge/3
  If/1 -> If Action Subsystem/Action

== system FaultCheck/FaultDiag_HighTask_100us/FltDetn/HWOverCurrDetn/HWOverCurrDetn/ErrCode ==
  ErrDetnFlgOut : Inport
  ErrCode : Inport  Port=2
  If : If  IfExpression=u1==0
  If Action Subsystem : Subsystem  TreatAsAtomicUnit=on
  If Action Subsystem1 : Subsystem  TreatAsAtomicUnit=on
  wires:
  ErrDetnFlgOut/1 -> If/1
  If/2 -> If Action Subsystem1/Action
  If/1 -> If Action Subsystem/Action
  ErrCode/1 -> If Action Subsystem1/1(ErrCod)

== system FaultCheck/FaultDiag_HighTask_100us/FltDetn/HWOverCurrDetn/HWOverCurrDetn/ErrDetn ==
  InputVal : Inport
  EnabDetn : Inport  Port=2
  ActvnDetn : Inport  Port=3
  ErrDeb : Inport  Port=4
  AND1 : Logic  AllPortsSameDT=off  OutDataTypeStr=boolean
  Constant10 : Constant  Value=FLT_ON
  Constant9 : Constant  Value=FLT_ON
  If : If  IfExpression=u1 == 0
  If Action Subsystem : Subsystem  TreatAsAtomicUnit=on
  If Action Subsystem1 : Subsystem  TreatAsAtomicUnit=on
  Merge : Merge
  Relational Operator3 : RelationalOperator  Operator===  OutDataTypeStr=boolean  RndMeth=Simplest  InputSameDT=off
  Relational Operator4 : RelationalOperator  Operator===  OutDataTypeStr=boolean  RndMeth=Simplest  InputSameDT=off
  Flt_HWOverCurrErrFlg : Outport
  wires:
  ErrDeb/1 -> If Action Subsystem1/2(ErrDeb)
  Merge/1 -> Flt_HWOverCurrErrFlg/1  "Flt_HWOverCurrErrFlg"
  If Action Subsystem/1(Out1) -> Merge/1
  If Action Subsystem1/1(Out1) -> Merge/2
  If/2 -> If Action Subsystem1/Action
  If/1 -> If Action Subsystem/Action
  AND1/1 -> If/1
  Relational Operator4/1 -> AND1/2
  Constant9/1 -> Relational Operator3/2
  Relational Operator3/1 -> AND1/1
  EnabDetn/1 -> Relational Operator4/2
  Constant10/1 -> Relational Operator4/1
  ActvnDetn/1 -> Relational Operator3/1
  InputVal/1 -> If Action Subsystem1/1(InputVal)

== system FaultCheck/FaultDiag_HighTask_100us/FltDetn/HWOverCurrDetn/HWOverCurrDetn/FltLvl ==
  ErrDetnFlgOut : Inport
  FltLvl : Inport  Port=2
  If : If  IfExpression=u1==0
  If Action Subsystem : Subsystem  TreatAsAtomicUnit=on
  If Action Subsystem1 : Subsystem  TreatAsAtomicUnit=on
  Merge : Merge
  Flt_HWOverCurrFltLvl : Outport
  wires:
  If Action Subsystem1/1(ValOut) -> Merge/2
  FltLvl/1 -> If Action Subsystem1/1(In)
  ErrDetnFlgOut/1 -> If/1
  If/2 -> If Action Subsystem1/Action
  If/1 -> If Action Subsystem/Action
  Merge/1 -> Flt_HWOverCurrFltLvl/1  "Flt_HWOverCurrFltLvl"
  If Action Subsystem/1(ValOut) -> Merge/1

== system FaultCheck/FaultDiag_HighTask_100us/FltDetn/HWOverCurrDetn/HWOverCurrDetn/Power Reduction Coefficient ==
  FltLvlOut : Inport
  PowRecCoef : Inport  Port=2
  If : If  IfExpression=u1<2  ElseIfExpressions=u1==2
  If Action Subsystem : Subsystem  TreatAsAtomicUnit=on
  If Action Subsystem1 : Subsystem  TreatAsAtomicUnit=on
  If Action Subsystem2 : Subsystem  TreatAsAtomicUnit=on
  Merge : Merge  Inputs=3
  Flt_HWOverCurrPowRecCoefOut : Outport
  wires:
  If/2 -> If Action Subsystem1/Action
  Merge/1 -> Flt_HWOverCurrPowRecCoefOut/1  "Flt_HWOverCurrPowRecCoefOut"
  If Action Subsystem/1(PowRecCoefOut) -> Merge/1
  If Action Subsystem1/1(PowRecCoefOut) -> Merge/2
  PowRecCoef/1 -> If Action Subsystem1/1(PowRecCoef)
  FltLvlOut/1 -> If/1
  If/3 -> If Action Subsystem2/Action
  If Action Subsystem2/1(PowRecCoefOut) -> Merge/3
  If/1 -> If Action Subsystem/Action

== system FaultCheck/FaultDiag_HighTask_100us/FltDetn/HWOverUdcDetn/HWOverCurrDetn/ErrCode ==
  ErrDetnFlgOut : Inport
  ErrCode : Inport  Port=2
  If : If  IfExpression=u1==0
  If Action Subsystem : Subsystem  TreatAsAtomicUnit=on
  If Action Subsystem1 : Subsystem  TreatAsAtomicUnit=on
  wires:
  ErrDetnFlgOut/1 -> If/1
  If/2 -> If Action Subsystem1/Action
  If/1 -> If Action Subsystem/Action
  ErrCode/1 -> If Action Subsystem1/1(ErrCod)

== system FaultCheck/FaultDiag_HighTask_100us/FltDetn/HWOverUdcDetn/HWOverCurrDetn/ErrDetn ==
  InputVal : Inport
  EnabDetn : Inport  Port=2
  ActvnDetn : Inport  Port=3
  ErrDeb : Inport  Port=4
  AND1 : Logic  AllPortsSameDT=off  OutDataTypeStr=boolean
  Constant10 : Constant  Value=FLT_ON
  Constant9 : Constant  Value=FLT_ON
  If : If  IfExpression=u1 == 0
  If Action Subsystem : Subsystem  TreatAsAtomicUnit=on
  If Action Subsystem1 : Subsystem  TreatAsAtomicUnit=on
  Merge : Merge
  Relational Operator3 : RelationalOperator  Operator===  OutDataTypeStr=boolean  RndMeth=Simplest  InputSameDT=off
  Relational Operator4 : RelationalOperator  Operator===  OutDataTypeStr=boolean  RndMeth=Simplest  InputSameDT=off
  Flt_HWOverUdcErrFlg : Outport
  wires:
  ErrDeb/1 -> If Action Subsystem1/2(ErrDeb)
  Merge/1 -> Flt_HWOverUdcErrFlg/1  "Flt_HWOverUdcErrFlg"
  If Action Subsystem/1(Out1) -> Merge/1
  If Action Subsystem1/1(Out1) -> Merge/2
  If/2 -> If Action Subsystem1/Action
  If/1 -> If Action Subsystem/Action
  AND1/1 -> If/1
  Relational Operator4/1 -> AND1/2
  Constant9/1 -> Relational Operator3/2
  Relational Operator3/1 -> AND1/1
  EnabDetn/1 -> Relational Operator4/2
  Constant10/1 -> Relational Operator4/1
  ActvnDetn/1 -> Relational Operator3/1
  InputVal/1 -> If Action Subsystem1/1(InputVal)

== system FaultCheck/FaultDiag_HighTask_100us/FltDetn/HWOverUdcDetn/HWOverCurrDetn/FltLvl ==
  ErrDetnFlgOut : Inport
  FltLvl : Inport  Port=2
  If : If  IfExpression=u1==0
  If Action Subsystem : Subsystem  TreatAsAtomicUnit=on
  If Action Subsystem1 : Subsystem  TreatAsAtomicUnit=on
  Merge : Merge
  Flt_HWOverUdcFltLvl : Outport
  wires:
  If Action Subsystem1/1(ValOut) -> Merge/2
  FltLvl/1 -> If Action Subsystem1/1(In)
  ErrDetnFlgOut/1 -> If/1
  If/2 -> If Action Subsystem1/Action
  If/1 -> If Action Subsystem/Action
  Merge/1 -> Flt_HWOverUdcFltLvl/1  "Flt_HWOverUdcFltLvl"
  If Action Subsystem/1(ValOut) -> Merge/1

== system FaultCheck/FaultDiag_HighTask_100us/FltDetn/HWOverUdcDetn/HWOverCurrDetn/Power Reduction Coefficient ==
  FltLvlOut : Inport
  PowRecCoef : Inport  Port=2
  If : If  IfExpression=u1<2  ElseIfExpressions=u1==2
  If Action Subsystem : Subsystem  TreatAsAtomicUnit=on
  If Action Subsystem1 : Subsystem  TreatAsAtomicUnit=on
  If Action Subsystem2 : Subsystem  TreatAsAtomicUnit=on
  Merge : Merge  Inputs=3
  Flt_HWOverUdcPowRecCoefOut : Outport
  wires:
  If/2 -> If Action Subsystem1/Action
  Merge/1 -> Flt_HWOverUdcPowRecCoefOut/1  "Flt_HWOverUdcPowRecCoefOut"
  If Action Subsystem/1(PowRecCoefOut) -> Merge/1
  If Action Subsystem1/1(PowRecCoefOut) -> Merge/2
  PowRecCoef/1 -> If Action Subsystem1/1(PowRecCoef)
  FltLvlOut/1 -> If/1
  If/3 -> If Action Subsystem2/Action
  If Action Subsystem2/1(PowRecCoefOut) -> Merge/3
  If/1 -> If Action Subsystem/Action

== system FaultCheck/FaultDiag_HighTask_100us/FltDetn/OverCurrDetn/Flt_IuOverCurrDetn/ErrCode1 ==
  ErrDetnFlgOut : Inport
  ErrCode : Inport  Port=2
  If : If  IfExpression=u1==0
  If Action Subsystem : Subsystem  TreatAsAtomicUnit=on
  If Action Subsystem1 : Subsystem  TreatAsAtomicUnit=on
  wires:
  ErrDetnFlgOut/1 -> If/1
  If/2 -> If Action Subsystem1/Action
  If/1 -> If Action Subsystem/Action
  ErrCode/1 -> If Action Subsystem1/1(ErrCod)

== system FaultCheck/FaultDiag_HighTask_100us/FltDetn/OverCurrDetn/Flt_IuOverCurrDetn/ErrDetn1 ==
  InputVal : Inport
  EnabDetn : Inport  Port=2
  ActvnDetn : Inport  Port=3
  HiLimPositv : Inport  Port=4
  HiLimNegatv : Inport  Port=5
  ErrDeb : Inport  Port=6
  AND1 : Logic  AllPortsSameDT=off  OutDataTypeStr=boolean
  Constant2 : Constant  Value=FLT_ON
  Constant3 : Constant  Value=FLT_ON
  If : If  IfExpression=u1 == 0
  If Action Subsystem : Subsystem  TreatAsAtomicUnit=on
  If Action Subsystem1 : Subsystem  TreatAsAtomicUnit=on
  Merge : Merge
  Relational Operator3 : RelationalOperator  Operator===  OutDataTypeStr=boolean  RndMeth=Simplest  InputSameDT=off
  Relational Operator4 : RelationalOperator  Operator===  OutDataTypeStr=boolean  RndMeth=Simplest  InputSameDT=off
  Flt_IuOverCurrErrDetnFlg : Outport
  wires:
  ErrDeb/1 -> If Action Subsystem1/2(ErrDeb)
  InputVal/1 -> If Action Subsystem1/1(InputVal)
  Merge/1 -> Flt_IuOverCurrErrDetnFlg/1  "Flt_IuOverCurrErrDetnFlg"
  If Action Subsystem/1(DetnFlg) -> Merge/1
  If Action Subsystem1/1(DetnFlg) -> Merge/2
  If/2 -> If Action Subsystem1/Action
  If/1 -> If Action Subsystem/Action
  AND1/1 -> If/1
  Relational Operator4/1 -> AND1/2
  Constant2/1 -> Relational Operator3/2
  Relational Operator3/1 -> AND1/1
  EnabDetn/1 -> Relational Operator4/2
  Constant3/1 -> Relational Operator4/1
  ActvnDetn/1 -> Relational Operator3/1
  HiLimPositv/1 -> If Action Subsystem1/3(HiLimPositv)
  HiLimNegatv/1 -> If Action Subsystem1/4(HiLimNegatv)

== system FaultCheck/FaultDiag_HighTask_100us/FltDetn/OverCurrDetn/Flt_IuOverCurrDetn/FltLvl ==
  ErrDetnFlgOut : Inport
  FltLvl : Inport  Port=2
  If : If  IfExpression=u1==0
  If Action Subsystem : Subsystem  TreatAsAtomicUnit=on
  If Action Subsystem1 : Subsystem  TreatAsAtomicUnit=on
  Merge : Merge
  Flt_IuOverCurrFltLvlOut : Outport
  wires:
  If Action Subsystem/1(ValOut) -> Merge/1
  Merge/1 -> Flt_IuOverCurrFltLvlOut/1  "Flt_IuOverCurrFltLvlOut"
  If/1 -> If Action Subsystem/Action
  If/2 -> If Action Subsystem1/Action
  ErrDetnFlgOut/1 -> If/1
  FltLvl/1 -> If Action Subsystem1/1(In)
  If Action Subsystem1/1(ValOut) -> Merge/2

== system FaultCheck/FaultDiag_HighTask_100us/FltDetn/OverCurrDetn/Flt_IuOverCurrDetn/Power Reduction Coefficient ==
  FltLvlOut : Inport
  PowRecCoef : Inport  Port=2
  If : If  IfExpression=u1<2  ElseIfExpressions=u1==2
  If Action Subsystem : Subsystem  TreatAsAtomicUnit=on
  If Action Subsystem1 : Subsystem  TreatAsAtomicUnit=on
  If Action Subsystem2 : Subsystem  TreatAsAtomicUnit=on
  Merge : Merge  Inputs=3
  Flt_IuOverCurrPowRecCoefOut : Outport
  wires:
  If/2 -> If Action Subsystem1/Action
  Merge/1 -> Flt_IuOverCurrPowRecCoefOut/1  "Flt_IuOverCurrPowRecCoefOut"
  If Action Subsystem/1(PowRecCoefOut) -> Merge/1
  If Action Subsystem1/1(PowRecCoefOut) -> Merge/2
  PowRecCoef/1 -> If Action Subsystem1/1(PowRecCoef)
  FltLvlOut/1 -> If/1
  If/3 -> If Action Subsystem2/Action
  If Action Subsystem2/1(PowRecCoefOut) -> Merge/3
  If/1 -> If Action Subsystem/Action

== system FaultCheck/FaultDiag_HighTask_100us/FltDetn/OverCurrDetn/Flt_IvOverCurrDetn/ErrCode1 ==
  ErrDetnFlgOut : Inport
  ErrCode : Inport  Port=2
  If : If  IfExpression=u1==0
  If Action Subsystem : Subsystem  TreatAsAtomicUnit=on
  If Action Subsystem1 : Subsystem  TreatAsAtomicUnit=on
  wires:
  ErrDetnFlgOut/1 -> If/1
  If/2 -> If Action Subsystem1/Action
  If/1 -> If Action Subsystem/Action
  ErrCode/1 -> If Action Subsystem1/1(ErrCod)

== system FaultCheck/FaultDiag_HighTask_100us/FltDetn/OverCurrDetn/Flt_IvOverCurrDetn/ErrDetn1 ==
  InputVal : Inport
  EnabDetn : Inport  Port=2
  ActvnDetn : Inport  Port=3
  UpLimPositv : Inport  Port=4
  UpLimNegatv : Inport  Port=5
  ErrDeb : Inport  Port=6
  AND1 : Logic  AllPortsSameDT=off  OutDataTypeStr=boolean
  Constant2 : Constant  Value=FLT_ON
  Constant3 : Constant  Value=FLT_ON
  If : If  IfExpression=u1 == 0
  If Action Subsystem : Subsystem  TreatAsAtomicUnit=on
  If Action Subsystem1 : Subsystem  TreatAsAtomicUnit=on
  Merge : Merge
  Relational Operator3 : RelationalOperator  Operator===  OutDataTypeStr=boolean  RndMeth=Simplest  InputSameDT=off
  Relational Operator4 : RelationalOperator  Operator===  OutDataTypeStr=boolean  RndMeth=Simplest  InputSameDT=off
  Flt_IvOverCurrErrDetnFlg : Outport  PortDimensions=1
  wires:
  UpLimNegatv/1 -> If Action Subsystem1/4(UpLimNegatv)
  UpLimPositv/1 -> If Action Subsystem1/3(UpLimPositv)
  ActvnDetn/1 -> Relational Operator3/1
  Constant3/1 -> Relational Operator4/1
  EnabDetn/1 -> Relational Operator4/2
  Relational Operator3/1 -> AND1/1
  Constant2/1 -> Relational Operator3/2
  Relational Operator4/1 -> AND1/2
  AND1/1 -> If/1
  If/1 -> If Action Subsystem/Action
  If/2 -> If Action Subsystem1/Action
  If Action Subsystem1/1(DetnFlg) -> Merge/2
  If Action Subsystem/1(DetnFlg) -> Merge/1
  Merge/1 -> Flt_IvOverCurrErrDetnFlg/1  "Flt_IvOverCurrErrDetnFlg"
  InputVal/1 -> If Action Subsystem1/1(InputVal)
  ErrDeb/1 -> If Action Subsystem1/2(ErrDeb)

== system FaultCheck/FaultDiag_HighTask_100us/FltDetn/OverCurrDetn/Flt_IvOverCurrDetn/FltLvl ==
  ErrDetnFlgOut : Inport
  FltLvl : Inport  Port=2
  If : If  IfExpression=u1==0
  If Action Subsystem : Subsystem  TreatAsAtomicUnit=on
  If Action Subsystem1 : Subsystem  TreatAsAtomicUnit=on
  Merge : Merge
  Flt_IvOverCurrFltLvlOut : Outport
  wires:
  If Action Subsystem1/1(ValOut) -> Merge/2
  FltLvl/1 -> If Action Subsystem1/1(In)
  ErrDetnFlgOut/1 -> If/1
  If/2 -> If Action Subsystem1/Action
  If/1 -> If Action Subsystem/Action
  Merge/1 -> Flt_IvOverCurrFltLvlOut/1  "Flt_IvOverCurrFltLvlOut"
  If Action Subsystem/1(ValOut) -> Merge/1

== system FaultCheck/FaultDiag_HighTask_100us/FltDetn/OverCurrDetn/Flt_IvOverCurrDetn/Power Reduction Coefficient ==
  FltLvlOut : Inport
  PowRecCoef : Inport  Port=2
  If : If  IfExpression=u1<2  ElseIfExpressions=u1==2
  If Action Subsystem : Subsystem  TreatAsAtomicUnit=on
  If Action Subsystem1 : Subsystem  TreatAsAtomicUnit=on
  If Action Subsystem2 : Subsystem  TreatAsAtomicUnit=on
  Merge : Merge  Inputs=3
  Flt_IvOverCurrPowRecCoefOut : Outport
  wires:
  Merge/1 -> Flt_IvOverCurrPowRecCoefOut/1  "Flt_IvOverCurrPowRecCoefOut"
  If Action Subsystem/1(PowRecCoefOut) -> Merge/1
  If Action Subsystem1/1(PowRecCoefOut) -> Merge/2
  PowRecCoef/1 -> If Action Subsystem1/1(PowRecCoef)
  FltLvlOut/1 -> If/1
  If Action Subsystem2/1(PowRecCoefOut) -> Merge/3
  If/1 -> If Action Subsystem/Action
  If/3 -> If Action Subsystem2/Action
  If/2 -> If Action Subsystem1/Action

== system FaultCheck/FaultDiag_HighTask_100us/FltDetn/OverCurrDetn/Flt_IwOverCurrDetn1/ErrCode1 ==
  ErrDetnFlgOut : Inport
  ErrCode : Inport  Port=2
  If : If  IfExpression=u1==0
  If Action Subsystem : Subsystem  TreatAsAtomicUnit=on
  If Action Subsystem1 : Subsystem  TreatAsAtomicUnit=on
  wires:
  ErrDetnFlgOut/1 -> If/1
  If/2 -> If Action Subsystem1/Action
  If/1 -> If Action Subsystem/Action
  ErrCode/1 -> If Action Subsystem1/1(ErrCod)

== system FaultCheck/FaultDiag_HighTask_100us/FltDetn/OverCurrDetn/Flt_IwOverCurrDetn1/ErrDetn1 ==
  InputVal : Inport
  EnabDetn : Inport  Port=2
  ActvnDetn : Inport  Port=3
  UpLimPositv : Inport  Port=4
  UpLimNegatv : Inport  Port=5
  ErrDeb : Inport  Port=6
  AND1 : Logic  AllPortsSameDT=off  OutDataTypeStr=boolean
  Constant2 : Constant  Value=FLT_ON
  Constant3 : Constant  Value=FLT_ON
  If : If  IfExpression=u1 == 0
  If Action Subsystem : Subsystem  TreatAsAtomicUnit=on
  If Action Subsystem1 : Subsystem  TreatAsAtomicUnit=on
  Merge : Merge
  Relational Operator3 : RelationalOperator  Operator===  OutDataTypeStr=boolean  RndMeth=Simplest  InputSameDT=off
  Relational Operator4 : RelationalOperator  Operator===  OutDataTypeStr=boolean  RndMeth=Simplest  InputSameDT=off
  Flt_IwOverCurrErrDetnFlg : Outport  PortDimensions=1
  wires:
  UpLimNegatv/1 -> If Action Subsystem1/4(UpLimNegatv)
  UpLimPositv/1 -> If Action Subsystem1/3(UpLimPositv)
  ActvnDetn/1 -> Relational Operator3/1
  Constant3/1 -> Relational Operator4/1
  EnabDetn/1 -> Relational Operator4/2
  Relational Operator3/1 -> AND1/1
  Constant2/1 -> Relational Operator3/2
  Relational Operator4/1 -> AND1/2
  AND1/1 -> If/1
  If/1 -> If Action Subsystem/Action
  If/2 -> If Action Subsystem1/Action
  If Action Subsystem1/1(DetnFlg) -> Merge/2
  If Action Subsystem/1(DetnFlg) -> Merge/1
  Merge/1 -> Flt_IwOverCurrErrDetnFlg/1  "Flt_IwOverCurrErrDetnFlg"
  InputVal/1 -> If Action Subsystem1/1(InputVal)
  ErrDeb/1 -> If Action Subsystem1/2(ErrDeb)

== system FaultCheck/FaultDiag_HighTask_100us/FltDetn/OverCurrDetn/Flt_IwOverCurrDetn1/FltLvl ==
  ErrDetnFlgOut : Inport
  FltLvl : Inport  Port=2
  If : If  IfExpression=u1==0
  If Action Subsystem : Subsystem  TreatAsAtomicUnit=on
  If Action Subsystem1 : Subsystem  TreatAsAtomicUnit=on
  Merge : Merge
  Flt_IwOverCurrFltLvlOut : Outport
  wires:
  If Action Subsystem1/1(ValOut) -> Merge/2
  FltLvl/1 -> If Action Subsystem1/1(In)
  ErrDetnFlgOut/1 -> If/1
  If/2 -> If Action Subsystem1/Action
  If/1 -> If Action Subsystem/Action
  Merge/1 -> Flt_IwOverCurrFltLvlOut/1  "Flt_IwOverCurrFltLvlOut"
  If Action Subsystem/1(ValOut) -> Merge/1

== system FaultCheck/FaultDiag_HighTask_100us/FltDetn/OverCurrDetn/Flt_IwOverCurrDetn1/Power Reduction Coefficient ==
  FltLvlOut : Inport
  PowRecCoef : Inport  Port=2
  If : If  IfExpression=u1<2  ElseIfExpressions=u1==2
  If Action Subsystem : Subsystem  TreatAsAtomicUnit=on
  If Action Subsystem1 : Subsystem  TreatAsAtomicUnit=on
  If Action Subsystem2 : Subsystem  TreatAsAtomicUnit=on
  Merge : Merge  Inputs=3
  Flt_IwOverCurrPowRecCoefOut : Outport
  wires:
  Merge/1 -> Flt_IwOverCurrPowRecCoefOut/1  "Flt_IwOverCurrPowRecCoefOut"
  If Action Subsystem/1(PowRecCoefOut) -> Merge/1
  If Action Subsystem1/1(PowRecCoefOut) -> Merge/2
  PowRecCoef/1 -> If Action Subsystem1/1(PowRecCoef)
  FltLvlOut/1 -> If/1
  If Action Subsystem2/1(PowRecCoefOut) -> Merge/3
  If/1 -> If Action Subsystem/Action
  If/3 -> If Action Subsystem2/Action
  If/2 -> If Action Subsystem1/Action

== system FaultCheck/FaultDiag_HighTask_100us/FltDetn/RecUDetn/RecUDetn/ErrCode1 ==
  note: SWFD--ComReq-01-13
  ErrDetnFlgOut : Inport
  ErrCode : Inport  Port=2
  If : If  IfExpression=u1==0
  If Action Subsystem : Subsystem  TreatAsAtomicUnit=on
  If Action Subsystem1 : Subsystem  TreatAsAtomicUnit=on
  wires:
  ErrCode/1 -> If Action Subsystem1/1(ErrCod)
  If/1 -> If Action Subsystem/Action
  If/2 -> If Action Subsystem1/Action
  ErrDetnFlgOut/1 -> If/1

== system FaultCheck/FaultDiag_HighTask_100us/FltDetn/RecUDetn/RecUDetn/ErrDetn ==
  InputVal : Inport
  EnabDetn : Inport  Port=2
  ActvnDetn : Inport  Port=3
  ErrDeb : Inport  Port=4
  AND1 : Logic  AllPortsSameDT=off  OutDataTypeStr=boolean
  Constant10 : Constant  Value=FLT_ON
  Constant9 : Constant  Value=FLT_ON
  If : If  IfExpression=u1 == 0
  If Action Subsystem : Subsystem  TreatAsAtomicUnit=on
  If Action Subsystem1 : Subsystem  TreatAsAtomicUnit=on
  Merge : Merge
  Relational Operator3 : RelationalOperator  Operator===  OutDataTypeStr=boolean  RndMeth=Simplest  InputSameDT=off
  Relational Operator4 : RelationalOperator  Operator===  OutDataTypeStr=boolean  RndMeth=Simplest  InputSameDT=off
  Flt_RecUErrFlg : Outport
  wires:
  ErrDeb/1 -> If Action Subsystem1/2(ErrDeb)
  InputVal/1 -> If Action Subsystem1/1(InputVal)
  Merge/1 -> Flt_RecUErrFlg/1  "Flt_RecUErrFlg"
  If Action Subsystem/1(Out1) -> Merge/1
  If Action Subsystem1/1(Out1) -> Merge/2
  If/2 -> If Action Subsystem1/Action
  If/1 -> If Action Subsystem/Action
  AND1/1 -> If/1
  Relational Operator4/1 -> AND1/2
  Constant9/1 -> Relational Operator3/2
  Relational Operator3/1 -> AND1/1
  EnabDetn/1 -> Relational Operator4/2
  Constant10/1 -> Relational Operator4/1
  ActvnDetn/1 -> Relational Operator3/1
